simulink model "P2_0D_model_parametrized"  (R2023a)
settings: Solver=ode4  StartTime=0.0  StopTime=inf  FixedStep=Ts  RelTol=1e-3
model workspace (MAT data in the model file):
  Ts = Simulink.Parameter
  Ts.Value = 0.0005
  Ts.DataType = 'auto'
  Ts.Complexity = 'real'
  Ts.Dimensions = [1 1]
undefined symbols (not defined in the file or in its folder): data, HR, left_ventricle_R_wall, MLAP, MRAP, openloop
libraries: Vessel x42, simulink x2
(part 1 of 2)
settings Model: Creator=emanuele  LastModifiedBy=priya
settings DataIOCC: FinalStateName=final_simstate  InitialState=new_simstate  SaveFinalState=on  SaveOperatingPoint=on
settings OptimizationCC: ReuseModelBlockBuffer=off

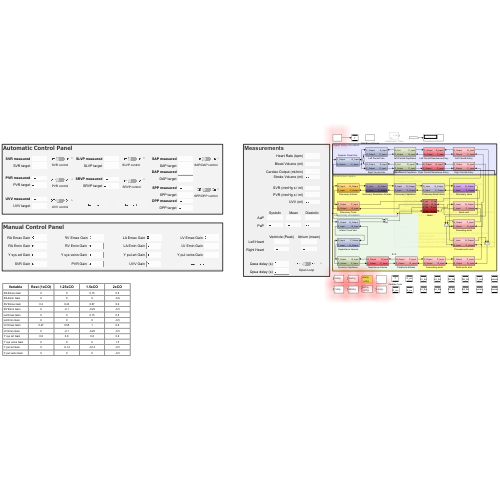
[thumbnail: Simulink's stored preview of the top-level diagram]
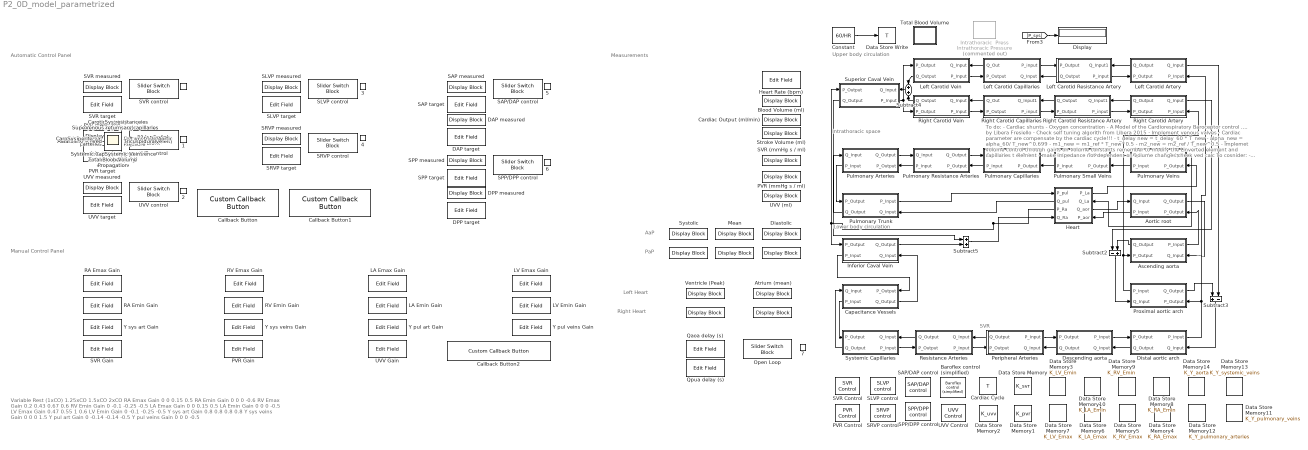
== system P2_0D_model_parametrized ==
  note: AaP
  note: Measurements
  note: Automatic Control Panel
  note: SVR
  note: To do:
      |
      | - Cardiac shunts
      | - Oxygen concentration
      | - A Model of the Cardiorespiratory  Baroceptor control .... by Libera Fresiello
      | - Check self tuning algorith from Libera 2015
      | - Implement venous valves
      | - Cardiac parameter are compensate by the cardiac cycle!!!
      |            - t_delay new = t_delay_60 * T_new
      |            - alpha_new = alpha_60/ T_new^0.699
      |            - m1_new = m1_ref * T_new^0.5
      |            - m2_new = m2_ref / T_new^0.5
      | - Implemet volume control through gains on volume constants
      | remember to modify the Linverted element and capillaries t element - make impedance
      | not dependent on volume changes
      |
      | check ved calc
      |
      | To cosnider:
      |
      | - Valves' Bernoulli resistance has to be divided by 100 or 1000. It strongly affects
      | the behaviour of the whole system
      | - The inductance and the resistances of the vessels do not change over time
      | - Reatime optimization  to patient ? like with smatwatch data (https://www.cardiacsense.com/wp-content/uploads/2019/10/2022_05_11_ENGLISH_WEBSITE.pdf).
      |
      | Ideas:
      |
      | - Patient specific optmisazion with smart watch, cloud server, etc foo prediction of???
      |   - High ematocrit level. Hypotension etc.
      | - Use locomotory data from patient during walking, incorporate it into the model,
      |   potentially demosntrate 1:1 coupling.
      | - maybe incorporate the metabolic consumpton too?
      | - Use MRI images of vasculature to derive geometrical parameters
      | - COmbine 0D model with 1 D model of specfic tract? check simvascular for ull ody model
      | - Black box for nils (protected model)
      |
      | Questions to Broomé:
      | - Do inductances and resistances change over time with vessel's radius?
      | - Having problem with allowing negative flow at the valves.
  note: Upper body circulation
  note: Intrathoracic space
  note: Lower body circulation
  note: Manual Control Panel
  note: PaP
  note: Left Heart
  note: Right Heart
  note: Variable
      | Rest (1xCO)
      | 1.25xCO
      | 1.5xCO
      | 2xCO
      |
      | RA Emax Gain
      | 0
      | 0
      | 0.15
      | 0.5
      |
      | RA Emin Gain
      | 0
      | 0
      | 0
      | -0.6
      |
      | RV Emax Gain
      | 0.2
      | 0.43
      | 0.67
      | 0.6
      |
      | RV Emin Gain
      | 0
      | -0.1
      | -0.25
      | -0.5
      |
      | LA Emax Gain
      | 0
      | 0
      | 0.15
      | 0.5
      |
      | LA Emin Gain
      | 0
      | 0
      | 0
      | -0.5
      |
      | LV Emax Gain
      | 0.47
      | 0.55
      | 1
      | 0.6
      |
      | LV Emin Gain
      | 0
      | -0.1
      | -0.25
      | -0.5
      |
      | Y sys art Gain
      | 0.8
      | 0.8
      | 0.8
      | 0.8
      |
      | Y sys veins Gain
      | 0
      | 0
      | 0
      | 1.5
      |
      | Y pul art Gain
      | 0
      | -0.14
      | -0.14
      | -0.5
      |
      | Y pul veins Gain
      | 0
      | 0
      | 0
      | -0.5
   {,3..7} (6 alike) : LampBlock  LabelPosition=Hide  Opacity=0.5
  "  " : DisplayBlock  LabelPosition=Hide  Format=Custom  Alignment=Left  Transparency=1  Layout=Fill available space  FormatString=%.2f
  "   " : DisplayBlock  LabelPosition=Hide  Format=Custom  Alignment=Left  Transparency=1  Layout=Fill available space  FormatString=%.2f
  "     " : DisplayBlock  LabelPosition=Hide  Format=Custom  Alignment=Left  Transparency=1  Layout=Fill available space  FormatString=%.2f
  "      " : DisplayBlock  LabelPosition=Hide  Format=Custom  Alignment=Left  Transparency=1  Layout=Fill available space  FormatString=%.2f
  "          " : DisplayBlock  LabelPosition=Hide  Format=Custom  Alignment=Left  Transparency=1  Layout=Fill available space  FormatString=%.2f
  " 1" : LampBlock  LabelPosition=Hide
  " 2" : LampBlock  LabelPosition=Hide
  Aortic root : Subsystem
      settings: PortSchema="{\"entries\":[{\"content\":{\"sides\":[{\"content\":{\"connectorIds\":[\"In1\",\"Out2\"]},\"type\":\"ConnectorPlacement.EquallySpacedRectSide\",\"uuid\":\"4620f5c1-12c0-4f29-952b-739216107ff5\"},{\"content\":{\"connectorIds\":[\"Out1\",\"In2\"],\"side\":\"RIGHT\"},\"type\":\"ConnectorPlacement.EquallySpacedRectSide\",\"uuid\":\"dda98628-74f0-4e08-ba9e-db399286a987\"},{\"content\":{\"connectorIds\":[],\"side\":\"TOP\"},\"type\":\"ConnectorPlacement.EquallySpacedRectSide\",\"uuid\":\"6ce998cb-1877-491b-b2c2-215d41cdcb23\"},{\"content\":{\"connectorIds\":[],\"side\":\"BOTTOM\"},\"type\":\"ConnectorPlacement.EquallySpacedRectSide\",\"uuid\":\"85207667-2600-4d53-af68-3471fed39a56\"}]},\"type\":\"ConnectorPlacement.EquallySpacedConnector\",\"uuid\":\"3b979ad0-f04d-4546-9a99-5921572b1183\"}],\"packageUris\":[\"http://schema.mathworks.com/mf0/Connector/R2020b\"],\"version\":\"1.0\"}"
  Ascending aorta : Subsystem  Description=asrwer
      settings: PortSchema="{\"entries\":[{\"content\":{\"sides\":[{\"content\":{\"connectorIds\":[\"Out2\",\"In1\"]},\"type\":\"ConnectorPlacement.EquallySpacedRectSide\",\"uuid\":\"4620f5c1-12c0-4f29-952b-739216107ff5\"},{\"content\":{\"connectorIds\":[\"Out1\",\"In2\"],\"side\":\"RIGHT\"},\"type\":\"ConnectorPlacement.EquallySpacedRectSide\",\"uuid\":\"dda98628-74f0-4e08-ba9e-db399286a987\"},{\"content\":{\"connectorIds\":[],\"side\":\"TOP\"},\"type\":\"ConnectorPlacement.EquallySpacedRectSide\",\"uuid\":\"6ce998cb-1877-491b-b2c2-215d41cdcb23\"},{\"content\":{\"connectorIds\":[],\"side\":\"BOTTOM\"},\"type\":\"ConnectorPlacement.EquallySpacedRectSide\",\"uuid\":\"dba296ee-e2cd-4942-9262-f71d521616c7\"}]},\"type\":\"ConnectorPlacement.EquallySpacedConnector\",\"uuid\":\"3b979ad0-f04d-4546-9a99-5921572b1183\"}],\"packageUris\":[\"http://schema.mathworks.com/mf0/Connector/R2020b\"],\"version\":\"1.0\"}"
  Atrium (mean) : DisplayBlock  LabelPosition=Hide  Format=Custom  Alignment=Left  Transparency=1  Layout=Fill available space  FormatString=%.2f
  Baroflex control (simplified) : Vessel/Baroflex control (simplified)  G_baro=0.04  P_target=92  T_target=60/72  onoff=off
      settings: SourceProductName=CVM
  Blood Volume (ml) : DisplayBlock  LabelPosition=Hide  Format=Custom  Alignment=Left  Transparency=1  Layout=Fill available space  FormatString=%.f
  Callback Button : CustomCallbackButton  Configuration="{\"components\":[{\"name\":\"BackgroundImageComponent\",\"settings\":{\"image\":{\"size\":[0,0],\"src\":\"default\",\"srcOrientation\":\"Right\"},\"position\":[0,0,1,1]}},{\"name\":\"ButtonStateComponent\",\"settings\":{\"buttonType\":\"momentary\",\"clickFcn\":\"coder.extrinsic('set_param')\\nset_param(['' bdroot '\\/SVR Control\\/Constant1'],'Value',sprintf('%d',0));\\nset_param(['' bdroot '\\/PVR Control\\/Constant1'],'Value',sprintf('%d',0));\\n\\nset_param(['' bdroot '\\/SLVP control\\/Constant1'],'Value',sprintf('%d',0));\\nset_param(['' bdroot '\\/SRVP control\\/Constant1'],'Value',sprintf('%d',0));\\n\\nset_param(['' bdroot '\\/SAP\\/\\/DAP control\\/Constant1'],'Value',sprintf('%d',0));\\nset_param(['' bdroot '\\/SPP\\/\\/DPP control\\/Constant1'],'Value',sprintf('%d',0));\\n\",\"onValue\":1,\"position\":[0,0,1,1],\"pressDelay\":\"500\",\"pressFcn\":\"\",\"repeatInterval\":\"0\",\"states\":[{\"horizontalAlignment\":\"center\",\"image\":{\"position\":[0,0,1,1],\"src\":\"default\",\"srcOrientation\":\"Right\"},\"label\":{\"color\":[0.01176470588,0.01176470588,0.01176470588,1],\"icon\":{\"size\":[0,0],\"src\":\"default\",\"srcOrientation\":\"Right\"},\"iconPlacement\":\"left\",\"text\":{\"content\":\"Turn off all\"}},\"labelOffset\":[0,0],\"verticalAlignment\":\"middle\"},{\"horizontalAlignment\":\"center\",\"image\":{\"position\":[0,0,1,1],\"src\":\"default\",\"srcOrientation\":\"Right\"},\"label\":{\"color\":[0.01176470588,0.01176470588,0.01176470588,1],\"icon\":{\"size\":[0,0],\"src\":\"default\",\"srcOrientation\":\"Right\"},\"iconPlacement\":\"left\",\"text\":{\"content\":\"Turn off all\"}},\"labelOffset\":[0,0],\"verticalAlignment\":\"middle\"},{\"horizontalAlignment\":\"center\",\"image\":{\"position\":[0,0,1,1],\"src\":\"default\",\"srcOrientation\":\"Right\"},\"label\":{\"color\":[0.01176470588,0.01176470588,0.01176470588,1],\"icon\":{\"size\":[0,0],\"src\":\"default\",\"srcOrientation\":\"Right\"},\"iconPlacement\":\"left\",\"text\":{\"content\":\"Turn off all\"}},\"labelOffset\":[0,0],\"verticalAlignment\":\"middle\"},{\"horizontalAlignment\":\"center\",\"image\":{\"position\":[0,0,1,1],\"src\":\"default\",\"srcOrientation\":\"Right\"},\"label\":{\"color\":[0.01176470588,0.01176470588,0.01176470588,1],\"icon\":{\"size\":[0,0],\"src\":\"default\",\"srcOrientation\":\"Right\"},\"iconPlacement\":\"left\",\"text\":{\"content\":\"Turn off all\"}},\"labelOffset\":[0,0],\"verticalAlignment\":\"middle\"}]}},{\"name\":\"ForegroundImageComponent\",\"settings\":{\"image\":{\"size\":[0,0],\"src\":\"default\",\"srcOrientation\":\"Right\"},\"isForeground\":1,\"position\":[0,0,1,1]}}],\"settings\":{\"BindingType\":\"standalone\",\"backgroundColor\":[244,244,244,1],\"backgroundOffset\":0.2,\"backgroundOpacity\":1,\"fixedAspectRatio\":\"off\",\"foregroundColor\":[0.01176470588,0.01176470588,0.01176470588,1],\"migratedFromLegacy\":true,\"useBackgroundColor\":true,\"variant\":\"callback\",\"version\":\"R2023a\"},\"type\":\"Button\"}"  CustomBackgroundColor="{\"color\":[0.9568627451,0.9568627451,0.9568627451],\"show\":true}"
  Callback Button1 : CustomCallbackButton  Configuration="{\"components\":[{\"name\":\"BackgroundImageComponent\",\"settings\":{\"image\":{\"size\":[0,0],\"src\":\"default\",\"srcOrientation\":\"Right\"},\"position\":[0,0,1,1]}},{\"name\":\"ButtonStateComponent\",\"settings\":{\"buttonType\":\"momentary\",\"clickFcn\":\"coder.extrinsic('set_param')\\nset_param(['' bdroot '\\/SVR Control\\/Constant1'],'Value',sprintf('%d',1));\\nset_param(['' bdroot '\\/PVR Control\\/Constant1'],'Value',sprintf('%d',1));\\n\\nset_param(['' bdroot '\\/SLVP control\\/Constant1'],'Value',sprintf('%d',1));\\nset_param(['' bdroot '\\/SRVP control\\/Constant1'],'Value',sprintf('%d',1));\\n\\nset_param(['' bdroot '\\/SAP\\/\\/DAP control\\/Constant1'],'Value',sprintf('%d',1));\\nset_param(['' bdroot '\\/SPP\\/\\/DPP control\\/Constant1'],'Value',sprintf('%d',1));\\n\",\"onValue\":1,\"position\":[0,0,1,1],\"pressDelay\":\"500\",\"pressFcn\":\"\",\"repeatInterval\":\"0\",\"states\":[{\"horizontalAlignment\":\"center\",\"image\":{\"position\":[0,0,1,1],\"src\":\"default\",\"srcOrientation\":\"Right\"},\"label\":{\"color\":[0.01176470588,0.01176470588,0.01176470588,1],\"icon\":{\"size\":[0,0],\"src\":\"default\",\"srcOrientation\":\"Right\"},\"iconPlacement\":\"left\",\"text\":{\"content\":\"Turn on all\"}},\"labelOffset\":[0,0],\"verticalAlignment\":\"middle\"},{\"horizontalAlignment\":\"center\",\"image\":{\"position\":[0,0,1,1],\"src\":\"default\",\"srcOrientation\":\"Right\"},\"label\":{\"color\":[0.01176470588,0.01176470588,0.01176470588,1],\"icon\":{\"size\":[0,0],\"src\":\"default\",\"srcOrientation\":\"Right\"},\"iconPlacement\":\"left\",\"text\":{\"content\":\"Turn on all\"}},\"labelOffset\":[0,0],\"verticalAlignment\":\"middle\"},{\"horizontalAlignment\":\"center\",\"image\":{\"position\":[0,0,1,1],\"src\":\"default\",\"srcOrientation\":\"Right\"},\"label\":{\"color\":[0.01176470588,0.01176470588,0.01176470588,1],\"icon\":{\"size\":[0,0],\"src\":\"default\",\"srcOrientation\":\"Right\"},\"iconPlacement\":\"left\",\"text\":{\"content\":\"Turn on all\"}},\"labelOffset\":[0,0],\"verticalAlignment\":\"middle\"},{\"horizontalAlignment\":\"center\",\"image\":{\"position\":[0,0,1,1],\"src\":\"default\",\"srcOrientation\":\"Right\"},\"label\":{\"color\":[0.01176470588,0.01176470588,0.01176470588,1],\"icon\":{\"size\":[0,0],\"src\":\"default\",\"srcOrientation\":\"Right\"},\"iconPlacement\":\"left\",\"text\":{\"content\":\"Turn on all\"}},\"labelOffset\":[0,0],\"verticalAlignment\":\"middle\"}]}},{\"name\":\"ForegroundImageComponent\",\"settings\":{\"image\":{\"size\":[0,0],\"src\":\"default\",\"srcOrientation\":\"Right\"},\"isForeground\":1,\"position\":[0,0,1,1]}}],\"settings\":{\"BindingType\":\"standalone\",\"backgroundColor\":[244,244,244,1],\"backgroundOffset\":0.2,\"backgroundOpacity\":1,\"fixedAspectRatio\":\"off\",\"foregroundColor\":[0.01176470588,0.01176470588,0.01176470588,1],\"migratedFromLegacy\":true,\"useBackgroundColor\":true,\"variant\":\"callback\",\"version\":\"R2023a\"},\"type\":\"Button\"}"  CustomBackgroundColor="{\"color\":[0.9568627451,0.9568627451,0.9568627451],\"show\":true}"
  Callback Button2 : CustomCallbackButton  Configuration="{\"components\":[{\"name\":\"BackgroundImageComponent\",\"settings\":{\"image\":{\"size\":[0,0],\"src\":\"default\",\"srcOrientation\":\"Right\"},\"position\":[0,0,1,1]}},{\"name\":\"ButtonStateComponent\",\"settings\":{\"buttonType\":\"momentary\",\"clickFcn\":\"coder.extrinsic('set_param')\\nset_param(['' bdroot '\\/SVR Control\\/K_svr'],'Value',sprintf('%d',0));\\nset_param(['' bdroot '\\/PVR Control\\/K_pvr'],'Value',sprintf('%d',0));\\n\\nset_param(['' bdroot '\\/SLVP control\\/K_LV_Emax'],'Value',sprintf('%d',0));\\nset_param(['' bdroot '\\/SLVP control\\/K_LV_Emin'],'Value',sprintf('%d',0));\\nset_param(['' bdroot '\\/SLVP control\\/K_LA_Emax'],'Value',sprintf('%d',0));\\nset_param(['' bdroot '\\/SLVP control\\/K_LA_Emin'],'Value',sprintf('%d',0));\\n\\nset_param(['' bdroot '\\/SRVP control\\/K_RV_Emax'],'Value',sprintf('%d',0));\\nset_param(['' bdroot '\\/SRVP control\\/K_RV_Emin'],'Value',sprintf('%d',0));\\nset_param(['' bdroot '\\/SRVP control\\/K_RA_Emax'],'Value',sprintf('%d',0));\\nset_param(['' bdroot '\\/SRVP control\\/K_RA_Emin'],'Value',sprintf('%d',0));\\n\\nset_param(['' bdroot '\\/SAP\\/\\/DAP control\\/K_Y_aorta'],'Value',sprintf('%d',0));\\nset_param(['' bdroot '\\/SAP\\/\\/DAP control\\/K_Y_systemic_veins'],'Value',sprintf('%d',0));\\n\\nset_param(['' bdroot '\\/SPP\\/\\/DPP control\\/K_Y_pulmonary_arteries'],'Value',sprintf('%d',0));\\nset_param(['' bdroot '\\/SPP\\/\\/DPP control\\/K_Y_pulmonary_veins'],'Value',sprintf('%d',0));\\n\\n\",\"onValue\":1,\"position\":[0,0,1,1],\"pressDelay\":\"500\",\"pressFcn\":\"\",\"repeatInterval\":\"0\",\"states\":[{\"horizontalAlignment\":\"center\",\"image\":{\"position\":[0,0,1,1],\"src\":\"default\",\"srcOrientation\":\"Right\"},\"label\":{\"color\":[0.01176470588,0.01176470588,0.01176470588,1],\"icon\":{\"size\":[0,0],\"src\":\"default\",\"srcOrientation\":\"Right\"},\"iconPlacement\":\"left\",\"text\":{\"content\":\"Reset Gains\"}},\"labelOffset\":[0,0],\"verticalAlignment\":\"middle\"},{\"horizontalAlignment\":\"center\",\"image\":{\"position\":[0,0,1,1],\"src\":\"default\",\"srcOrientation\":\"Right\"},\"label\":{\"color\":[0.01176470588,0.01176470588,0.01176470588,1],\"icon\":{\"size\":[0,0],\"src\":\"default\",\"srcOrientation\":\"Right\"},\"iconPlacement\":\"left\",\"text\":{\"content\":\"Reset Gains\"}},\"labelOffset\":[0,0],\"verticalAlignment\":\"middle\"},{\"horizontalAlignment\":\"center\",\"image\":{\"position\":[0,0,1,1],\"src\":\"default\",\"srcOrientation\":\"Right\"},\"label\":{\"color\":[0.01176470588,0.01176470588,0.01176470588,1],\"icon\":{\"size\":[0,0],\"src\":\"default\",\"srcOrientation\":\"Right\"},\"iconPlacement\":\"left\",\"text\":{\"content\":\"Reset Gains\"}},\"labelOffset\":[0,0],\"verticalAlignment\":\"middle\"},{\"horizontalAlignment\":\"center\",\"image\":{\"position\":[0,0,1,1],\"src\":\"default\",\"srcOrientation\":\"Right\"},\"label\":{\"color\":[0.01176470588,0.01176470588,0.01176470588,1],\"icon\":{\"size\":[0,0],\"src\":\"default\",\"srcOrientation\":\"Right\"},\"iconPlacement\":\"left\",\"text\":{\"content\":\"Reset Gains\"}},\"labelOffset\":[0,0],\"verticalAlignment\":\"middle\"}]}},{\"name\":\"ForegroundImageComponent\",\"settings\":{\"image\":{\"size\":[0,0],\"src\":\"default\",\"srcOrientation\":\"Right\"},\"isForeground\":1,\"position\":[0,0,1,1]}}],\"settings\":{\"BindingType\":\"standalone\",\"backgroundColor\":[244,244,244,1],\"backgroundOffset\":0.2,\"backgroundOpacity\":1,\"fixedAspectRatio\":\"off\",\"foregroundColor\":[0.01176470588,0.01176470588,0.01176470588,1],\"migratedFromLegacy\":true,\"useBackgroundColor\":true,\"variant\":\"callback\",\"version\":\"R2023a\"},\"type\":\"Button\"}"  CustomBackgroundColor="{\"color\":[0.9568627451,0.9568627451,0.9568627451],\"show\":true}"
  Capacitance Vessels : Subsystem  Description=asrwer
      settings: PortSchema="{\"entries\":[{\"content\":{\"sides\":[{\"content\":{\"connectorIds\":[\"In1\",\"Out2\"]},\"type\":\"ConnectorPlacement.EquallySpacedRectSide\",\"uuid\":\"4620f5c1-12c0-4f29-952b-739216107ff5\"},{\"content\":{\"connectorIds\":[\"In2\",\"Out1\"],\"side\":\"RIGHT\"},\"type\":\"ConnectorPlacement.EquallySpacedRectSide\",\"uuid\":\"dda98628-74f0-4e08-ba9e-db399286a987\"},{\"content\":{\"connectorIds\":[],\"side\":\"TOP\"},\"type\":\"ConnectorPlacement.EquallySpacedRectSide\",\"uuid\":\"6ce998cb-1877-491b-b2c2-215d41cdcb23\"},{\"content\":{\"connectorIds\":[],\"side\":\"BOTTOM\"},\"type\":\"ConnectorPlacement.EquallySpacedRectSide\",\"uuid\":\"722bc419-c275-4c63-b409-b29152115373\"}]},\"type\":\"ConnectorPlacement.EquallySpacedConnector\",\"uuid\":\"3b979ad0-f04d-4546-9a99-5921572b1183\"}],\"packageUris\":[\"http://schema.mathworks.com/mf0/Connector/R2020b\"],\"version\":\"1.0\"}"
  Cardiac Cycle : DataStoreMemory  DataStoreName=T  WriteAfterWriteMsg=warning  InitialValue=1  ShowAdditionalParam=off  OutMin=0  OutMax=1000
  Cardiac Output (ml/min) : DisplayBlock  LabelPosition=Hide  Format=Custom  Alignment=Left  Transparency=1  Layout=Fill available space  FormatString=%.f
  Constant : Constant  Value=60/HR
  DAP measured : DisplayBlock  LabelPosition=Hide  Format=Custom  Alignment=Left  Transparency=1  Layout=Fill available space  FormatString=%.2f
  DAP target : EditField  LabelPosition=Hide  ShowInitialText=on  Alignment=Left
  DPP measured : DisplayBlock  LabelPosition=Hide  Format=Custom  Alignment=Left  Transparency=1  Layout=Fill available space  FormatString=%.2f
  DPP target : EditField  LabelPosition=Hide  ShowInitialText=on  Alignment=Left
  Data Store Memory : DataStoreMemory  DataStoreName=K_svr  WriteAfterWriteMsg=warning  ShowAdditionalParam=off
  Data Store Memory1 : DataStoreMemory  DataStoreName=K_pvr  WriteAfterWriteMsg=warning  ShowAdditionalParam=off
  Data Store Memory10 : DataStoreMemory  DataStoreName=K_LA_Emin  WriteAfterWriteMsg=warning  ShowAdditionalParam=off
  Data Store Memory11 : DataStoreMemory  DataStoreName=K_Y_pulmonary_veins  WriteAfterWriteMsg=warning  ShowAdditionalParam=off
  Data Store Memory12 : DataStoreMemory  DataStoreName=K_Y_pulmonary_arteries  WriteAfterWriteMsg=warning  ShowAdditionalParam=off
  Data Store Memory13 : DataStoreMemory  DataStoreName=K_Y_systemic_veins  WriteAfterWriteMsg=warning  ShowAdditionalParam=off
  Data Store Memory14 : DataStoreMemory  DataStoreName=K_Y_aorta  WriteAfterWriteMsg=warning  ShowAdditionalParam=off
  Data Store Memory2 : DataStoreMemory  DataStoreName=K_uvv  WriteAfterWriteMsg=warning  ShowAdditionalParam=off
  Data Store Memory3 : DataStoreMemory  DataStoreName=K_LV_Emin  WriteAfterWriteMsg=warning  ShowAdditionalParam=off
  Data Store Memory4 : DataStoreMemory  DataStoreName=K_RA_Emax  WriteAfterWriteMsg=warning  ShowAdditionalParam=off
  Data Store Memory5 : DataStoreMemory  DataStoreName=K_RV_Emax  WriteAfterWriteMsg=warning  ShowAdditionalParam=off
  Data Store Memory6 : DataStoreMemory  DataStoreName=K_LA_Emax  WriteAfterWriteMsg=warning  ShowAdditionalParam=off
  Data Store Memory7 : DataStoreMemory  DataStoreName=K_LV_Emax  WriteAfterWriteMsg=warning  ShowAdditionalParam=off
  Data Store Memory8 : DataStoreMemory  DataStoreName=K_RA_Emin  WriteAfterWriteMsg=warning  ShowAdditionalParam=off
  Data Store Memory9 : DataStoreMemory  DataStoreName=K_RV_Emin  WriteAfterWriteMsg=warning  ShowAdditionalParam=off
  Data Store Write : DataStoreWrite  DataStoreName=T  IndexOptions=Index vector (dialog)  Indices=1  OutputSizes=1
  Descending aorta : Subsystem  Description=asrwer
      settings: PortSchema="{\"entries\":[{\"content\":{\"sides\":[{\"content\":{\"connectorIds\":[\"In1\",\"Out2\"]},\"type\":\"ConnectorPlacement.EquallySpacedRectSide\",\"uuid\":\"4620f5c1-12c0-4f29-952b-739216107ff5\"},{\"content\":{\"connectorIds\":[\"Out1\",\"In2\"],\"side\":\"RIGHT\"},\"type\":\"ConnectorPlacement.EquallySpacedRectSide\",\"uuid\":\"dda98628-74f0-4e08-ba9e-db399286a987\"},{\"content\":{\"connectorIds\":[],\"side\":\"TOP\"},\"type\":\"ConnectorPlacement.EquallySpacedRectSide\",\"uuid\":\"6ce998cb-1877-491b-b2c2-215d41cdcb23\"},{\"content\":{\"connectorIds\":[],\"side\":\"BOTTOM\"},\"type\":\"ConnectorPlacement.EquallySpacedRectSide\",\"uuid\":\"98e366c2-00e2-468b-b3a5-0ce1b16c883f\"}]},\"type\":\"ConnectorPlacement.EquallySpacedConnector\",\"uuid\":\"3b979ad0-f04d-4546-9a99-5921572b1183\"}],\"packageUris\":[\"http://schema.mathworks.com/mf0/Connector/R2020b\"],\"version\":\"1.0\"}"
  Diastolic : DisplayBlock  LabelPosition=Hide  Format=Custom  Alignment=Left  Transparency=1  Layout=Fill available space  FormatString=%.2f
  Display : Display
  Distal aortic arch : Subsystem  Description=asrwer
      settings: PortSchema="{\"entries\":[{\"content\":{\"sides\":[{\"content\":{\"connectorIds\":[\"In1\",\"Out2\"]},\"type\":\"ConnectorPlacement.EquallySpacedRectSide\",\"uuid\":\"4620f5c1-12c0-4f29-952b-739216107ff5\"},{\"content\":{\"connectorIds\":[\"Out1\",\"In2\"],\"side\":\"RIGHT\"},\"type\":\"ConnectorPlacement.EquallySpacedRectSide\",\"uuid\":\"dda98628-74f0-4e08-ba9e-db399286a987\"},{\"content\":{\"connectorIds\":[],\"side\":\"TOP\"},\"type\":\"ConnectorPlacement.EquallySpacedRectSide\",\"uuid\":\"6ce998cb-1877-491b-b2c2-215d41cdcb23\"},{\"content\":{\"connectorIds\":[],\"side\":\"BOTTOM\"},\"type\":\"ConnectorPlacement.EquallySpacedRectSide\",\"uuid\":\"1f1286b1-33d8-470d-99d1-3841bccf9133\"}]},\"type\":\"ConnectorPlacement.EquallySpacedConnector\",\"uuid\":\"3b979ad0-f04d-4546-9a99-5921572b1183\"}],\"packageUris\":[\"http://schema.mathworks.com/mf0/Connector/R2020b\"],\"version\":\"1.0\"}"
  Heart : Subsystem  Description=asrwer
      settings: PortSchema="{\"entries\":[{\"content\":{\"sides\":[{\"content\":{\"connectorIds\":[\"In1\",\"Out3\",\"Out4\",\"In2\"]},\"type\":\"ConnectorPlacement.EquallySpacedRectSide\",\"uuid\":\"95824f71-698a-4f4d-a993-6df26fe534d7\"},{\"content\":{\"connectorIds\":[\"Out1\",\"In3\",\"Out2\",\"In4\"],\"side\":\"RIGHT\"},\"type\":\"ConnectorPlacement.EquallySpacedRectSide\",\"uuid\":\"a8959a41-c68c-4f70-a35f-cb85dc600e61\"},{\"content\":{\"connectorIds\":[],\"side\":\"TOP\"},\"type\":\"ConnectorPlacement.EquallySpacedRectSide\",\"uuid\":\"0158d717-51c0-4653-88b6-d7632d8acf9b\"},{\"content\":{\"connectorIds\":[],\"side\":\"BOTTOM\"},\"type\":\"ConnectorPlacement.EquallySpacedRectSide\",\"uuid\":\"36b7b652-46be-43bf-a0da-22ec9d4b557c\"}]},\"type\":\"ConnectorPlacement.EquallySpacedConnector\",\"uuid\":\"7f917747-c70e-4597-9ded-e790c0b0e5f8\"}],\"packageUris\":[\"http://schema.mathworks.com/mf0/Connector/R2020b\"],\"version\":\"1.0\"}"
  Heart Rate (bpm) : EditField  LabelPosition=Hide  ShowInitialText=on  Alignment=Left
  Inferior Caval Vein : Subsystem  Description=asrwer
      settings: PortSchema="{\"entries\":[{\"content\":{\"sides\":[{\"content\":{\"connectorIds\":[\"In1\",\"Out2\"]},\"type\":\"ConnectorPlacement.EquallySpacedRectSide\",\"uuid\":\"4620f5c1-12c0-4f29-952b-739216107ff5\"},{\"content\":{\"connectorIds\":[\"Out1\",\"In2\"],\"side\":\"RIGHT\"},\"type\":\"ConnectorPlacement.EquallySpacedRectSide\",\"uuid\":\"dda98628-74f0-4e08-ba9e-db399286a987\"},{\"content\":{\"connectorIds\":[],\"side\":\"TOP\"},\"type\":\"ConnectorPlacement.EquallySpacedRectSide\",\"uuid\":\"6ce998cb-1877-491b-b2c2-215d41cdcb23\"},{\"content\":{\"connectorIds\":[],\"side\":\"BOTTOM\"},\"type\":\"ConnectorPlacement.EquallySpacedRectSide\",\"uuid\":\"6fb320e2-add0-4ab2-8fb4-43aaa029b4e4\"}]},\"type\":\"ConnectorPlacement.EquallySpacedConnector\",\"uuid\":\"3b979ad0-f04d-4546-9a99-5921572b1183\"}],\"packageUris\":[\"http://schema.mathworks.com/mf0/Connector/R2020b\"],\"version\":\"1.0\"}"
  Intrathoracic  Press : Vessel/Intrathoracic Pressure  Commented=on  t_ins=2  t_exp=3  p_ita=1.8  p_itb=-5.5
      settings: SourceProductName=CVM
  LA Emax Gain : EditField  LabelPosition=Hide  ShowInitialText=on  Alignment=Left
  LA Emin Gain : EditField  LabelPosition=Hide  ShowInitialText=on  Alignment=Left
  LV Emax Gain : EditField  LabelPosition=Hide  ShowInitialText=on  Alignment=Left
  LV Emin Gain : EditField  LabelPosition=Hide  ShowInitialText=on  Alignment=Left
  Left Carotid Artery : Subsystem  Description=asrwer
      settings: PortSchema="{\"entries\":[{\"content\":{\"sides\":[{\"content\":{\"connectorIds\":[\"Out2\",\"In1\"]},\"type\":\"ConnectorPlacement.EquallySpacedRectSide\",\"uuid\":\"4620f5c1-12c0-4f29-952b-739216107ff5\"},{\"content\":{\"connectorIds\":[\"Out1\",\"In2\"],\"side\":\"RIGHT\"},\"type\":\"ConnectorPlacement.EquallySpacedRectSide\",\"uuid\":\"dda98628-74f0-4e08-ba9e-db399286a987\"},{\"content\":{\"connectorIds\":[],\"side\":\"TOP\"},\"type\":\"ConnectorPlacement.EquallySpacedRectSide\",\"uuid\":\"6ce998cb-1877-491b-b2c2-215d41cdcb23\"},{\"content\":{\"connectorIds\":[],\"side\":\"BOTTOM\"},\"type\":\"ConnectorPlacement.EquallySpacedRectSide\",\"uuid\":\"47027a70-0169-4a10-9704-3eebb5be1f94\"}]},\"type\":\"ConnectorPlacement.EquallySpacedConnector\",\"uuid\":\"3b979ad0-f04d-4546-9a99-5921572b1183\"}],\"packageUris\":[\"http://schema.mathworks.com/mf0/Connector/R2020b\"],\"version\":\"1.0\"}"
  Left Carotid Capillaries : Subsystem  Description=asrwer
      settings: PortSchema="{\"entries\":[{\"content\":{\"sides\":[{\"content\":{\"connectorIds\":[\"Out2\",\"In1\"]},\"type\":\"ConnectorPlacement.EquallySpacedRectSide\",\"uuid\":\"4620f5c1-12c0-4f29-952b-739216107ff5\"},{\"content\":{\"connectorIds\":[\"Out1\",\"In2\"],\"side\":\"RIGHT\"},\"type\":\"ConnectorPlacement.EquallySpacedRectSide\",\"uuid\":\"dda98628-74f0-4e08-ba9e-db399286a987\"},{\"content\":{\"connectorIds\":[],\"side\":\"TOP\"},\"type\":\"ConnectorPlacement.EquallySpacedRectSide\",\"uuid\":\"6ce998cb-1877-491b-b2c2-215d41cdcb23\"},{\"content\":{\"connectorIds\":[],\"side\":\"BOTTOM\"},\"type\":\"ConnectorPlacement.EquallySpacedRectSide\",\"uuid\":\"55c6bb06-9ed0-4db0-b546-e99e0ef08408\"}]},\"type\":\"ConnectorPlacement.EquallySpacedConnector\",\"uuid\":\"3b979ad0-f04d-4546-9a99-5921572b1183\"}],\"packageUris\":[\"http://schema.mathworks.com/mf0/Connector/R2020b\"],\"version\":\"1.0\"}"
  Left Carotid Resistance Artery : Subsystem  Description=asrwer
      settings: PortSchema="{\"entries\":[{\"content\":{\"sides\":[{\"content\":{\"connectorIds\":[\"In1\",\"Out2\"]},\"type\":\"ConnectorPlacement.EquallySpacedRectSide\",\"uuid\":\"d2373093-dd34-4525-a7d5-a44f41a4186f\"},{\"content\":{\"connectorIds\":[\"In2\",\"Out1\"],\"side\":\"RIGHT\"},\"type\":\"ConnectorPlacement.EquallySpacedRectSide\",\"uuid\":\"d0ccba4c-fde8-4729-94ab-e77f6e90fb41\"},{\"content\":{\"connectorIds\":[],\"side\":\"TOP\"},\"type\":\"ConnectorPlacement.EquallySpacedRectSide\",\"uuid\":\"7f992dfa-60d0-4d20-a39d-6e17177f43eb\"},{\"content\":{\"connectorIds\":[],\"side\":\"BOTTOM\"},\"type\":\"ConnectorPlacement.EquallySpacedRectSide\",\"uuid\":\"2327e57f-2f10-4013-b93e-75b24ceebb4e\"}]},\"type\":\"ConnectorPlacement.EquallySpacedConnector\",\"uuid\":\"d7eff068-f330-41b8-9147-abcbffe8f160\"}],\"packageUris\":[\"http://schema.mathworks.com/mf0/Connector/R2020b\"],\"version\":\"1.0\"}"
  Left Carotid Vein : Subsystem  Description=asrwer
      settings: PortSchema="{\"entries\":[{\"content\":{\"sides\":[{\"content\":{\"connectorIds\":[\"In1\",\"Out2\"]},\"type\":\"ConnectorPlacement.EquallySpacedRectSide\",\"uuid\":\"4620f5c1-12c0-4f29-952b-739216107ff5\"},{\"content\":{\"connectorIds\":[\"In2\",\"Out1\"],\"side\":\"RIGHT\"},\"type\":\"ConnectorPlacement.EquallySpacedRectSide\",\"uuid\":\"dda98628-74f0-4e08-ba9e-db399286a987\"},{\"content\":{\"connectorIds\":[],\"side\":\"TOP\"},\"type\":\"ConnectorPlacement.EquallySpacedRectSide\",\"uuid\":\"6ce998cb-1877-491b-b2c2-215d41cdcb23\"}]},\"type\":\"ConnectorPlacement.EquallySpacedConnector\",\"uuid\":\"3b979ad0-f04d-4546-9a99-5921572b1183\"}],\"packageUris\":[\"http://schema.mathworks.com/mf0/Connector/R2020b\"],\"version\":\"1.0\"}"
  Mean : DisplayBlock  LabelPosition=Hide  Format=Custom  Alignment=Left  Transparency=1  Layout=Fill available space  FormatString=%.2f
  Open Loop : SliderSwitchBlock  LabelPosition=Hide
      settings: Values={{'Off', 'On'}, [0 1]}
  PVR (mmHg s / ml) : DisplayBlock  LabelPosition=Hide  Format=Custom  Alignment=Left  Transparency=1  Layout=Fill available space  FormatString=%.2f
  PVR Control : Vessel/PVR Control  PVR_0=PVR  onoff=off
      link override Constant1: Value=0
      link override K_pvr: Value=0
      link override PID Controller: P=0.2  I=0.2
      settings: SourceProductName=CVM
  PVR Gain : EditField  LabelPosition=Hide  ShowInitialText=on  Alignment=Left
  PVR control : SliderSwitchBlock  LabelPosition=Hide
      settings: Values={{'Off', 'On'}, [0 1]}
  PVR measured : DisplayBlock  LabelPosition=Hide  Format=Custom  Alignment=Left  Transparency=1  Layout=Fill available space  FormatString=%.2f
  PVR target : EditField  LabelPosition=Hide  ShowInitialText=on  Alignment=Left
  Peripheral Arteries : Subsystem  Description=asrwer
      settings: PortSchema="{\"entries\":[{\"content\":{\"sides\":[{\"content\":{\"connectorIds\":[\"Out2\",\"In1\"]},\"type\":\"ConnectorPlacement.EquallySpacedRectSide\",\"uuid\":\"4620f5c1-12c0-4f29-952b-739216107ff5\"},{\"content\":{\"connectorIds\":[\"Out1\",\"In2\"],\"side\":\"RIGHT\"},\"type\":\"ConnectorPlacement.EquallySpacedRectSide\",\"uuid\":\"dda98628-74f0-4e08-ba9e-db399286a987\"},{\"content\":{\"connectorIds\":[],\"side\":\"TOP\"},\"type\":\"ConnectorPlacement.EquallySpacedRectSide\",\"uuid\":\"6ce998cb-1877-491b-b2c2-215d41cdcb23\"}]},\"type\":\"ConnectorPlacement.EquallySpacedConnector\",\"uuid\":\"3b979ad0-f04d-4546-9a99-5921572b1183\"}],\"packageUris\":[\"http://schema.mathworks.com/mf0/Connector/R2020b\"],\"version\":\"1.0\"}"
  Proximal aortic arch : Subsystem  Description=asrwer
      settings: PortSchema="{\"entries\":[{\"content\":{\"sides\":[{\"content\":{\"connectorIds\":[\"Out2\",\"In1\"]},\"type\":\"ConnectorPlacement.EquallySpacedRectSide\",\"uuid\":\"4620f5c1-12c0-4f29-952b-739216107ff5\"},{\"content\":{\"connectorIds\":[\"Out1\",\"In2\"],\"side\":\"RIGHT\"},\"type\":\"ConnectorPlacement.EquallySpacedRectSide\",\"uuid\":\"dda98628-74f0-4e08-ba9e-db399286a987\"},{\"content\":{\"connectorIds\":[],\"side\":\"TOP\"},\"type\":\"ConnectorPlacement.EquallySpacedRectSide\",\"uuid\":\"6ce998cb-1877-491b-b2c2-215d41cdcb23\"},{\"content\":{\"connectorIds\":[],\"side\":\"BOTTOM\"},\"type\":\"ConnectorPlacement.EquallySpacedRectSide\",\"uuid\":\"6fdba645-d59c-41ca-a267-e7525d3dc150\"}]},\"type\":\"ConnectorPlacement.EquallySpacedConnector\",\"uuid\":\"3b979ad0-f04d-4546-9a99-5921572b1183\"}],\"packageUris\":[\"http://schema.mathworks.com/mf0/Connector/R2020b\"],\"version\":\"1.0\"}"
  Pulmonary Arteries : Subsystem  Description=asrwer
      settings: PortSchema="{\"entries\":[{\"content\":{\"sides\":[{\"content\":{\"connectorIds\":[\"In1\",\"Out2\"]},\"type\":\"ConnectorPlacement.EquallySpacedRectSide\",\"uuid\":\"4620f5c1-12c0-4f29-952b-739216107ff5\"},{\"content\":{\"connectorIds\":[\"Out1\",\"In2\"],\"side\":\"RIGHT\"},\"type\":\"ConnectorPlacement.EquallySpacedRectSide\",\"uuid\":\"dda98628-74f0-4e08-ba9e-db399286a987\"},{\"content\":{\"connectorIds\":[],\"side\":\"TOP\"},\"type\":\"ConnectorPlacement.EquallySpacedRectSide\",\"uuid\":\"6ce998cb-1877-491b-b2c2-215d41cdcb23\"},{\"content\":{\"connectorIds\":[],\"side\":\"BOTTOM\"},\"type\":\"ConnectorPlacement.EquallySpacedRectSide\",\"uuid\":\"b2958bd4-f048-459f-a2a1-00e3322b7fc4\"}]},\"type\":\"ConnectorPlacement.EquallySpacedConnector\",\"uuid\":\"3b979ad0-f04d-4546-9a99-5921572b1183\"}],\"packageUris\":[\"http://schema.mathworks.com/mf0/Connector/R2020b\"],\"version\":\"1.0\"}"
  Pulmonary Capillaries : Subsystem  Description=asrwer
      settings: PortSchema="{\"entries\":[{\"content\":{\"sides\":[{\"content\":{\"connectorIds\":[\"In1\",\"Out2\"]},\"type\":\"ConnectorPlacement.EquallySpacedRectSide\",\"uuid\":\"4620f5c1-12c0-4f29-952b-739216107ff5\"},{\"content\":{\"connectorIds\":[\"Out1\",\"In2\"],\"side\":\"RIGHT\"},\"type\":\"ConnectorPlacement.EquallySpacedRectSide\",\"uuid\":\"dda98628-74f0-4e08-ba9e-db399286a987\"},{\"content\":{\"connectorIds\":[],\"side\":\"TOP\"},\"type\":\"ConnectorPlacement.EquallySpacedRectSide\",\"uuid\":\"6ce998cb-1877-491b-b2c2-215d41cdcb23\"},{\"content\":{\"connectorIds\":[],\"side\":\"BOTTOM\"},\"type\":\"ConnectorPlacement.EquallySpacedRectSide\",\"uuid\":\"a5d17b15-fcf6-4394-a6ba-03d04e8a34a2\"}]},\"type\":\"ConnectorPlacement.EquallySpacedConnector\",\"uuid\":\"3b979ad0-f04d-4546-9a99-5921572b1183\"}],\"packageUris\":[\"http://schema.mathworks.com/mf0/Connector/R2020b\"],\"version\":\"1.0\"}"
  Pulmonary Resistance Arteries : Subsystem  Description=asrwer
      settings: PortSchema="{\"entries\":[{\"content\":{\"sides\":[{\"content\":{\"connectorIds\":[\"In1\",\"Out2\"]},\"type\":\"ConnectorPlacement.EquallySpacedRectSide\",\"uuid\":\"4620f5c1-12c0-4f29-952b-739216107ff5\"},{\"content\":{\"connectorIds\":[\"Out1\",\"In2\"],\"side\":\"RIGHT\"},\"type\":\"ConnectorPlacement.EquallySpacedRectSide\",\"uuid\":\"dda98628-74f0-4e08-ba9e-db399286a987\"},{\"content\":{\"connectorIds\":[],\"side\":\"TOP\"},\"type\":\"ConnectorPlacement.EquallySpacedRectSide\",\"uuid\":\"6ce998cb-1877-491b-b2c2-215d41cdcb23\"},{\"content\":{\"connectorIds\":[],\"side\":\"BOTTOM\"},\"type\":\"ConnectorPlacement.EquallySpacedRectSide\",\"uuid\":\"a4fcb2d7-d0b3-4cd9-b62c-2f8a41b0f34e\"}]},\"type\":\"ConnectorPlacement.EquallySpacedConnector\",\"uuid\":\"3b979ad0-f04d-4546-9a99-5921572b1183\"}],\"packageUris\":[\"http://schema.mathworks.com/mf0/Connector/R2020b\"],\"version\":\"1.0\"}"
  Pulmonary Small Veins : Subsystem  Description=asrwer
      settings: PortSchema="{\"entries\":[{\"content\":{\"sides\":[{\"content\":{\"connectorIds\":[\"In1\",\"Out2\"]},\"type\":\"ConnectorPlacement.EquallySpacedRectSide\",\"uuid\":\"4620f5c1-12c0-4f29-952b-739216107ff5\"},{\"content\":{\"connectorIds\":[\"Out1\",\"In2\"],\"side\":\"RIGHT\"},\"type\":\"ConnectorPlacement.EquallySpacedRectSide\",\"uuid\":\"dda98628-74f0-4e08-ba9e-db399286a987\"},{\"content\":{\"connectorIds\":[],\"side\":\"TOP\"},\"type\":\"ConnectorPlacement.EquallySpacedRectSide\",\"uuid\":\"6ce998cb-1877-491b-b2c2-215d41cdcb23\"},{\"content\":{\"connectorIds\":[],\"side\":\"BOTTOM\"},\"type\":\"ConnectorPlacement.EquallySpacedRectSide\",\"uuid\":\"137012d7-11b1-4b2c-ba99-c13cd95b2b50\"}]},\"type\":\"ConnectorPlacement.EquallySpacedConnector\",\"uuid\":\"3b979ad0-f04d-4546-9a99-5921572b1183\"}],\"packageUris\":[\"http://schema.mathworks.com/mf0/Connector/R2020b\"],\"version\":\"1.0\"}"
  Pulmonary Trunk : Subsystem  Description=asrwer
      settings: PortSchema="{\"entries\":[{\"content\":{\"sides\":[{\"content\":{\"connectorIds\":[\"In1\",\"Out2\"]},\"type\":\"ConnectorPlacement.EquallySpacedRectSide\",\"uuid\":\"4620f5c1-12c0-4f29-952b-739216107ff5\"},{\"content\":{\"connectorIds\":[\"Out1\",\"In2\"],\"side\":\"RIGHT\"},\"type\":\"ConnectorPlacement.EquallySpacedRectSide\",\"uuid\":\"dda98628-74f0-4e08-ba9e-db399286a987\"},{\"content\":{\"connectorIds\":[],\"side\":\"TOP\"},\"type\":\"ConnectorPlacement.EquallySpacedRectSide\",\"uuid\":\"6ce998cb-1877-491b-b2c2-215d41cdcb23\"},{\"content\":{\"connectorIds\":[],\"side\":\"BOTTOM\"},\"type\":\"ConnectorPlacement.EquallySpacedRectSide\",\"uuid\":\"04da4d59-f989-4121-a1c1-6ca6c24a4d8d\"}]},\"type\":\"ConnectorPlacement.EquallySpacedConnector\",\"uuid\":\"3b979ad0-f04d-4546-9a99-5921572b1183\"}],\"packageUris\":[\"http://schema.mathworks.com/mf0/Connector/R2020b\"],\"version\":\"1.0\"}"
  Pulmonary Veins : Subsystem  Description=asrwer
      settings: PortSchema="{\"entries\":[{\"content\":{\"sides\":[{\"content\":{\"connectorIds\":[\"In1\",\"Out2\"]},\"type\":\"ConnectorPlacement.EquallySpacedRectSide\",\"uuid\":\"4620f5c1-12c0-4f29-952b-739216107ff5\"},{\"content\":{\"connectorIds\":[\"Out1\",\"In2\"],\"side\":\"RIGHT\"},\"type\":\"ConnectorPlacement.EquallySpacedRectSide\",\"uuid\":\"dda98628-74f0-4e08-ba9e-db399286a987\"},{\"content\":{\"connectorIds\":[],\"side\":\"TOP\"},\"type\":\"ConnectorPlacement.EquallySpacedRectSide\",\"uuid\":\"6ce998cb-1877-491b-b2c2-215d41cdcb23\"},{\"content\":{\"connectorIds\":[],\"side\":\"BOTTOM\"},\"type\":\"ConnectorPlacement.EquallySpacedRectSide\",\"uuid\":\"3a23e96a-9068-4331-9d6b-a32064471a48\"}]},\"type\":\"ConnectorPlacement.EquallySpacedConnector\",\"uuid\":\"3b979ad0-f04d-4546-9a99-5921572b1183\"}],\"packageUris\":[\"http://schema.mathworks.com/mf0/Connector/R2020b\"],\"version\":\"1.0\"}"
  Qaoa delay (s) : EditField  LabelPosition=Hide  ShowInitialText=on  Alignment=Left
  Qpua delay (s) : EditField  LabelPosition=Hide  ShowInitialText=on  Alignment=Left
  RA Emax Gain : EditField  LabelPosition=Hide  ShowInitialText=on  Alignment=Left
  RA Emin Gain : EditField  LabelPosition=Hide  ShowInitialText=on  Alignment=Left
  RV Emax Gain : EditField  LabelPosition=Hide  ShowInitialText=on  Alignment=Left
  RV Emin Gain : EditField  LabelPosition=Hide  ShowInitialText=on  Alignment=Left
  Resistance Arteries : Subsystem  Description=asrwer
      settings: PortSchema="{\"entries\":[{\"content\":{\"sides\":[{\"content\":{\"connectorIds\":[\"In1\",\"Out2\"]},\"type\":\"ConnectorPlacement.EquallySpacedRectSide\",\"uuid\":\"4620f5c1-12c0-4f29-952b-739216107ff5\"},{\"content\":{\"connectorIds\":[\"Out1\",\"In2\"],\"side\":\"RIGHT\"},\"type\":\"ConnectorPlacement.EquallySpacedRectSide\",\"uuid\":\"dda98628-74f0-4e08-ba9e-db399286a987\"},{\"content\":{\"connectorIds\":[],\"side\":\"TOP\"},\"type\":\"ConnectorPlacement.EquallySpacedRectSide\",\"uuid\":\"6ce998cb-1877-491b-b2c2-215d41cdcb23\"},{\"content\":{\"connectorIds\":[],\"side\":\"BOTTOM\"},\"type\":\"ConnectorPlacement.EquallySpacedRectSide\",\"uuid\":\"1ab5c822-e7a5-49ea-823d-95e461b1ff07\"}]},\"type\":\"ConnectorPlacement.EquallySpacedConnector\",\"uuid\":\"3b979ad0-f04d-4546-9a99-5921572b1183\"}],\"packageUris\":[\"http://schema.mathworks.com/mf0/Connector/R2020b\"],\"version\":\"1.0\"}"
  Right Carotid Artery : Subsystem  Description=asrwer
      settings: PortSchema="{\"entries\":[{\"content\":{\"sides\":[{\"content\":{\"connectorIds\":[\"Out2\",\"In1\"]},\"type\":\"ConnectorPlacement.EquallySpacedRectSide\",\"uuid\":\"4620f5c1-12c0-4f29-952b-739216107ff5\"},{\"content\":{\"connectorIds\":[\"Out1\",\"In2\"],\"side\":\"RIGHT\"},\"type\":\"ConnectorPlacement.EquallySpacedRectSide\",\"uuid\":\"dda98628-74f0-4e08-ba9e-db399286a987\"},{\"content\":{\"connectorIds\":[],\"side\":\"TOP\"},\"type\":\"ConnectorPlacement.EquallySpacedRectSide\",\"uuid\":\"6ce998cb-1877-491b-b2c2-215d41cdcb23\"},{\"content\":{\"connectorIds\":[],\"side\":\"BOTTOM\"},\"type\":\"ConnectorPlacement.EquallySpacedRectSide\",\"uuid\":\"5d964695-aedc-48ec-816e-6d149f9baa1a\"}]},\"type\":\"ConnectorPlacement.EquallySpacedConnector\",\"uuid\":\"3b979ad0-f04d-4546-9a99-5921572b1183\"}],\"packageUris\":[\"http://schema.mathworks.com/mf0/Connector/R2020b\"],\"version\":\"1.0\"}"
  Right Carotid Capillaries : Subsystem  Description=asrwer
      settings: PortSchema="{\"entries\":[{\"content\":{\"sides\":[{\"content\":{\"connectorIds\":[\"Out2\",\"In1\"]},\"type\":\"ConnectorPlacement.EquallySpacedRectSide\",\"uuid\":\"4620f5c1-12c0-4f29-952b-739216107ff5\"},{\"content\":{\"connectorIds\":[\"In2\",\"Out1\"],\"side\":\"RIGHT\"},\"type\":\"ConnectorPlacement.EquallySpacedRectSide\",\"uuid\":\"dda98628-74f0-4e08-ba9e-db399286a987\"},{\"content\":{\"connectorIds\":[],\"side\":\"TOP\"},\"type\":\"ConnectorPlacement.EquallySpacedRectSide\",\"uuid\":\"6ce998cb-1877-491b-b2c2-215d41cdcb23\"},{\"content\":{\"connectorIds\":[],\"side\":\"BOTTOM\"},\"type\":\"ConnectorPlacement.EquallySpacedRectSide\",\"uuid\":\"cace3d24-f2c5-4b3d-b351-04ba56070658\"}]},\"type\":\"ConnectorPlacement.EquallySpacedConnector\",\"uuid\":\"3b979ad0-f04d-4546-9a99-5921572b1183\"}],\"packageUris\":[\"http://schema.mathworks.com/mf0/Connector/R2020b\"],\"version\":\"1.0\"}"
  Right Carotid Resistance Artery : Subsystem  Description=asrwer
      settings: PortSchema="{\"entries\":[{\"content\":{\"sides\":[{\"content\":{\"connectorIds\":[\"Out2\",\"In1\"]},\"type\":\"ConnectorPlacement.EquallySpacedRectSide\",\"uuid\":\"4620f5c1-12c0-4f29-952b-739216107ff5\"},{\"content\":{\"connectorIds\":[\"In2\",\"Out1\"],\"side\":\"RIGHT\"},\"type\":\"ConnectorPlacement.EquallySpacedRectSide\",\"uuid\":\"dda98628-74f0-4e08-ba9e-db399286a987\"},{\"content\":{\"connectorIds\":[],\"side\":\"TOP\"},\"type\":\"ConnectorPlacement.EquallySpacedRectSide\",\"uuid\":\"6ce998cb-1877-491b-b2c2-215d41cdcb23\"},{\"content\":{\"connectorIds\":[],\"side\":\"BOTTOM\"},\"type\":\"ConnectorPlacement.EquallySpacedRectSide\",\"uuid\":\"f6d8c471-30f5-492c-bb7b-f051effd3cec\"}]},\"type\":\"ConnectorPlacement.EquallySpacedConnector\",\"uuid\":\"3b979ad0-f04d-4546-9a99-5921572b1183\"}],\"packageUris\":[\"http://schema.mathworks.com/mf0/Connector/R2020b\"],\"version\":\"1.0\"}"
  Right Carotid Vein : Subsystem  Description=asrwer
      settings: PortSchema="{\"entries\":[{\"content\":{\"sides\":[{\"content\":{\"connectorIds\":[\"Out2\",\"In1\"]},\"type\":\"ConnectorPlacement.EquallySpacedRectSide\",\"uuid\":\"4620f5c1-12c0-4f29-952b-739216107ff5\"},{\"content\":{\"connectorIds\":[\"In2\",\"Out1\"],\"side\":\"RIGHT\"},\"type\":\"ConnectorPlacement.EquallySpacedRectSide\",\"uuid\":\"dda98628-74f0-4e08-ba9e-db399286a987\"},{\"content\":{\"connectorIds\":[],\"side\":\"TOP\"},\"type\":\"ConnectorPlacement.EquallySpacedRectSide\",\"uuid\":\"6ce998cb-1877-491b-b2c2-215d41cdcb23\"}]},\"type\":\"ConnectorPlacement.EquallySpacedConnector\",\"uuid\":\"3b979ad0-f04d-4546-9a99-5921572b1183\"}],\"packageUris\":[\"http://schema.mathworks.com/mf0/Connector/R2020b\"],\"version\":\"1.0\"}"
  SAP measured : DisplayBlock  LabelPosition=Hide  Format=Custom  Alignment=Left  Transparency=1  Layout=Fill available space  FormatString=%.2f
  SAP target : EditField  LabelPosition=Hide  ShowInitialText=on  Alignment=Left
  SAP/DAP control : Vessel/SAP//DAP control  SAP_0=SAP  DAP_0=DAP  dt=0.1  onoff=off
      link override Constant1: Value=0
      link override K_Y_aorta: Value=0
      link override K_Y_systemic_veins: Value=0
      link override PID Controller: UpperSaturationLimit=5
      settings: SourceProductName=CVM
  "SAP/DAP control " : SliderSwitchBlock  LabelPosition=Hide
      settings: Values={{'Off', 'On'}, [0 1]}
  SLVP control : Vessel/SLVP control  SLVP_0=MAP  dt=1  onoff=off
      link override Constant1: Value=0
      link override K_LA_Emax: Value=0
      link override K_LA_Emin: Value=0
      link override K_LV_Emax: Value=0
      link override K_LV_Emin: Value=0
      link override PID Controller: P=0.01  I=0.01  UpperSaturationLimit=5
      settings: LibrarySourceBlock=Vessel/SAP control  SourceProductName=CVM
  "SLVP control  " : SliderSwitchBlock  LabelPosition=Hide
      settings: Values={{'Off', 'On'}, [0 1]}
  SLVP measured : DisplayBlock  LabelPosition=Hide  Format=Custom  Alignment=Left  Transparency=1  Layout=Fill available space  FormatString=%.2f
  SLVP target : EditField  LabelPosition=Hide  ShowInitialText=on  Alignment=Left
  SPP measured : DisplayBlock  LabelPosition=Hide  Format=Custom  Alignment=Left  Transparency=1  Layout=Fill available space  FormatString=%.2f
  SPP target : EditField  LabelPosition=Hide  ShowInitialText=on  Alignment=Left
  SPP/DPP control : Vessel/SPP//DPP control  SPP_0=SPP  DPP_0=DPP  dt=0.1  onoff=off
      link override Constant1: Value=0
      link override K_Y_pulmonary_arteries: Value=0
      link override K_Y_pulmonary_veins: Value=0
      link override PID Controller: P=0.01  I=0.01  UpperSaturationLimit=5
      settings: SourceProductName=CVM
  "SPP/DPP control " : SliderSwitchBlock  LabelPosition=Hide
      settings: Values={{'Off', 'On'}, [0 1]}
  SRVP control : Vessel/SRVP control  SRVP_0=MPP  dt=1  onoff=off
      link override Constant1: Value=0
      link override K_RA_Emax: Value=0
      link override K_RA_Emin: Value=0
      link override K_RV_Emax: Value=0
      link override K_RV_Emin: Value=0
      link override PID Controller: P=0.01  I=0.01  UpperSaturationLimit=6
      settings: LibrarySourceBlock=Vessel/SPP control1  SourceProductName=CVM
  "SRVP control " : SliderSwitchBlock  LabelPosition=Hide
      settings: Values={{'Off', 'On'}, [0 1]}
  SRVP measured : DisplayBlock  LabelPosition=Hide  Format=Custom  Alignment=Left  Transparency=1  Layout=Fill available space  FormatString=%.2f
  SRVP target : EditField  LabelPosition=Hide  ShowInitialText=on  Alignment=Left
  SVR (mmHg s / ml) : DisplayBlock  LabelPosition=Hide  Format=Custom  Alignment=Left  Transparency=1  Layout=Fill available space  FormatString=%.2f
  SVR Control : Vessel/SVR Control  SVR_0=SVR  onoff=off
      link override Constant1: Value=0
      link override K_svr: Value=0
      settings: SourceProductName=CVM
  SVR Gain : EditField  LabelPosition=Hide  ShowInitialText=on  Alignment=Left
  SVR control : SliderSwitchBlock  LabelPosition=Hide
      settings: Values={{'Off', 'On'}, [0 1]}
  SVR measured : DisplayBlock  LabelPosition=Hide  Format=Custom  Alignment=Left  Transparency=1  Layout=Fill available space  FormatString=%.2f
  SVR target : EditField  LabelPosition=Hide  ShowInitialText=on  Alignment=Left
  Stroke Volume (ml) : DisplayBlock  LabelPosition=Hide  Format=Custom  Alignment=Left  Transparency=1  Layout=Fill available space  FormatString=%.2f
  Subtract2 : Sum  Inputs=-+
  Subtract3 : Sum  Inputs=+-
  Subtract4 : Sum
  Subtract5 : Sum
  Superior Caval Vein : Subsystem  Description=asrwer
      settings: PortSchema="{\"entries\":[{\"content\":{\"sides\":[{\"content\":{\"connectorIds\":[\"In1\",\"Out2\"]},\"type\":\"ConnectorPlacement.EquallySpacedRectSide\",\"uuid\":\"4620f5c1-12c0-4f29-952b-739216107ff5\"},{\"content\":{\"connectorIds\":[\"In2\",\"Out1\"],\"side\":\"RIGHT\"},\"type\":\"ConnectorPlacement.EquallySpacedRectSide\",\"uuid\":\"dda98628-74f0-4e08-ba9e-db399286a987\"},{\"content\":{\"connectorIds\":[],\"side\":\"TOP\"},\"type\":\"ConnectorPlacement.EquallySpacedRectSide\",\"uuid\":\"6ce998cb-1877-491b-b2c2-215d41cdcb23\"},{\"content\":{\"connectorIds\":[],\"side\":\"BOTTOM\"},\"type\":\"ConnectorPlacement.EquallySpacedRectSide\",\"uuid\":\"5f47a899-ed05-43b2-ba58-6d035433b88e\"}]},\"type\":\"ConnectorPlacement.EquallySpacedConnector\",\"uuid\":\"3b979ad0-f04d-4546-9a99-5921572b1183\"}],\"packageUris\":[\"http://schema.mathworks.com/mf0/Connector/R2020b\"],\"version\":\"1.0\"}"
  "Systemic Capillaries " : Subsystem  Description=asrwer
      settings: PortSchema="{\"entries\":[{\"content\":{\"sides\":[{\"content\":{\"connectorIds\":[\"In1\",\"Out2\"]},\"type\":\"ConnectorPlacement.EquallySpacedRectSide\",\"uuid\":\"4620f5c1-12c0-4f29-952b-739216107ff5\"},{\"content\":{\"connectorIds\":[\"In2\",\"Out1\"],\"side\":\"RIGHT\"},\"type\":\"ConnectorPlacement.EquallySpacedRectSide\",\"uuid\":\"dda98628-74f0-4e08-ba9e-db399286a987\"},{\"content\":{\"connectorIds\":[],\"side\":\"TOP\"},\"type\":\"ConnectorPlacement.EquallySpacedRectSide\",\"uuid\":\"6ce998cb-1877-491b-b2c2-215d41cdcb23\"},{\"content\":{\"connectorIds\":[],\"side\":\"BOTTOM\"},\"type\":\"ConnectorPlacement.EquallySpacedRectSide\",\"uuid\":\"621182d5-32aa-4c84-a747-47e09e96be96\"}]},\"type\":\"ConnectorPlacement.EquallySpacedConnector\",\"uuid\":\"3b979ad0-f04d-4546-9a99-5921572b1183\"}],\"packageUris\":[\"http://schema.mathworks.com/mf0/Connector/R2020b\"],\"version\":\"1.0\"}"
  Systolic : DisplayBlock  LabelPosition=Hide  Format=Custom  Alignment=Left  Transparency=1  Layout=Fill available space  FormatString=%.2f
  Total Blood Volume : Subsystem
  UVV (ml) : DisplayBlock  LabelPosition=Hide  Format=Custom  Alignment=Left  Transparency=1  Layout=Fill available space  FormatString=%.2f
  UVV Control : Vessel/UVV Control  UVV_0=UVV  onoff=off
      link override Constant1: Value=0
      link override K_uvv: Value=0
      link override PID Controller: I=0.001
      link override PID Controller1: LowerSaturationLimit=-0.95  P=0.001  I=0.001
      settings: SourceProductName=CVM
  UVV Gain : EditField  LabelPosition=Hide  ShowInitialText=on  Alignment=Left
  UVV control : SliderSwitchBlock  LabelPosition=Hide
      settings: Values={{'Off', 'On'}, [0 1]}
  UVV measured : DisplayBlock  LabelPosition=Hide  Format=Custom  Alignment=Left  Transparency=1  Layout=Fill available space  FormatString=%.2f
  UVV target : EditField  LabelPosition=Hide  ShowInitialText=on  Alignment=Left
  Ventricle (Peak) : DisplayBlock  LabelPosition=Hide  Format=Custom  Alignment=Left  Transparency=1  Layout=Fill available space  FormatString=%.2f
  Y pul art Gain : EditField  LabelPosition=Hide  ShowInitialText=on  Alignment=Left
  Y pul veins Gain : EditField  LabelPosition=Hide  ShowInitialText=on  Alignment=Left
  Y sys art Gain : EditField  LabelPosition=Hide  ShowInitialText=on  Alignment=Left
  Y sys veins Gain : EditField  LabelPosition=Hide  ShowInitialText=on  Alignment=Left
  Aorta (ascending) : Scope
  Aorta (descending) : Scope
  Aorta (distal) : Scope
  Aorta (proxima) : Scope
  Aorta (root) : Scope
  Aortic Valve : Scope
  Aplysia graphs : Scope
  Baroflex control : Scope
  Cardiac Output control : Scope
  Carotid Artery (left) : Scope
  Carotid Artery (right) : Scope
  Carotid Capillaries (left) : Scope
  Carotid Capillaries (right) : Scope
  Carotid resistance Artery (right) : Scope
  Carotid veins (right) : Scope
  Coronary Resistance Artery (right) : Scope
  Coronary arteries flow : Scope
  Elastances : Scope
  Heart Pressures : Scope
  Heart Volume : Scope
  Impedance convergence : Scope
  Inferior Vena cava : Scope
  Intrathoracic pressure : Scope
  Left ventricle/Aortic Pressure : Scope
  Mitral Valve : Scope
  Pressure Wave Propagation : Scope
  Pulmonary Valve : Scope
  Pulmonary capillaries : Scope
  R/ Atrium : Scope
  Scope{,1..6} (7 alike) : Scope
  Superior Vena cava : Scope
  Sys perifereal arteries : Scope
  Sys resistance arteries : Scope
  Systemic Capillaries : Scope
  Systemic Veins : Scope
  Total Bloob Volume : Scope
  Tricuspid Valve : Scope
  Ved : Scope
  Venous return : Scope
  wires:
  Pulmonary Trunk/2("Q_Output ") -> Pulmonary Arteries/1(Q_Input)
  Pulmonary Arteries/2("P_Input ") -> Pulmonary Trunk/1(P_Output)
  Pulmonary Arteries/1("Q_Output ") -> Pulmonary Resistance Arteries/1(Q_Input)
  Pulmonary Resistance Arteries/2("P_Input ") -> Pulmonary Arteries/2(P_Output)
  Pulmonary Resistance Arteries/1("Q_Output ") -> Pulmonary Capillaries/1(Q_Input)
  Pulmonary Capillaries/2("P_Input ") -> Pulmonary Resistance Arteries/2(P_Output)
  Pulmonary Capillaries/1("Q_Output ") -> Pulmonary Small Veins/1(Q_Input)
  Pulmonary Small Veins/2("P_Input ") -> Pulmonary Capillaries/2(P_Output)
  Pulmonary Small Veins/1("Q_Output ") -> Pulmonary Veins/1(Q_Input)
  Pulmonary Veins/2("P_Input ") -> Pulmonary Small Veins/2(P_Output)
  Aortic root/1("Q_Output ") -> Ascending aorta/2(Q_Input)
  Ascending aorta/1("P_Input ") -> Aortic root/2(P_Output)
  Ascending aorta/2("Q_Output ") -> Subtract2/2
  Proximal aortic arch/2("P_Input ") -> Ascending aorta/1(P_Output), Right Carotid Artery/2(P_Input)
  Proximal aortic arch/1("Q_Output ") -> Subtract3/1
  Distal aortic arch/2("Q_Output ") -> Descending aorta/2(Q_Input)
  Descending aorta/1("P_Input ") -> Distal aortic arch/1(P_Output)
  Peripheral Arteries/1("P_Input ") -> Descending aorta/1(P_Output)
  Descending aorta/2("Q_Output ") -> Peripheral Arteries/2(Q_Input)
  Peripheral Arteries/2("Q_Output ") -> Resistance Arteries/1(Q_Input)
  Resistance Arteries/2("P_Input ") -> Peripheral Arteries/1(P_Output)
  Resistance Arteries/1("Q_Output ") -> "Systemic Capillaries "/2(Q_Input)
  "Systemic Capillaries "/1("P_Input ") -> Resistance Arteries/2(P_Output)
  "Systemic Capillaries "/2("Q_Output ") -> Capacitance Vessels/1(Q_Input)
  Capacitance Vessels/2("P_Input ") -> "Systemic Capillaries "/1(P_Output)
  Inferior Caval Vein/1("P_Input ") -> Capacitance Vessels/2(P_Output)
  Capacitance Vessels/1("Q_Output ") -> Inferior Caval Vein/1(Q_Input)
  Right Carotid Artery/1(Q_Input) -> Subtract2/1
  Subtract2/1 -> Proximal aortic arch/1(Q_Input)
  Subtract3/1 -> Distal aortic arch/2(Q_Input)
  Left Carotid Artery/1(Q_Input) -> Subtract3/2
  Distal aortic arch/1("P_Input ") -> Proximal aortic arch/2(P_Output), Left Carotid Artery/2(P_Input)
  Left Carotid Capillaries/2(Q_Out) -> Left Carotid Vein/2(Q_Input)
  Left Carotid Vein/1("P_Input ") -> Left Carotid Capillaries/1(P_Output)
  Right Carotid Capillaries/2(Q_Out) -> Right Carotid Vein/2(Q_Input)
  Right Carotid Vein/1("P_Input ") -> Right Carotid Capillaries/1(P_Output)
  Superior Caval Vein/2("P_Input ") -> Left Carotid Vein/1(P_Output), Right Carotid Vein/1(P_Output)
  Subtract4/1 -> Superior Caval Vein/1(Q_Input)
  Right Carotid Vein/2("Q_Output ") -> Subtract4/2
  Left Carotid Vein/2("Q_Output ") -> Subtract4/1
  Inferior Caval Vein/2("Q_Output ") -> Subtract5/2
  Superior Caval Vein/1("Q_Output ") -> Subtract5/1
  Subtract5/1 -> Heart/2(Q_Ra)
  Heart/3(Q_pul) -> Pulmonary Trunk/2(Q_Input)
  Heart/2(Q_aor) -> Aortic root/1(Q_Input)
  Aortic root/2("P_Input ") -> Heart/4(P_aor)
  Pulmonary Trunk/1("P_Input ") -> Heart/1(P_pul)
  Pulmonary Veins/1("Q_Output ") -> Heart/3(Q_La)
  Heart/1(P_La) -> Pulmonary Veins/2(P_Output)
  Heart/4(P_Ra) -> Superior Caval Vein/2(P_Output), Inferior Caval Vein/2(P_Output)
  Left Carotid Capillaries/1(P_input) -> Left Carotid Resistance Artery/1(P_Output)
  Left Carotid Resistance Artery/2(Q_Output) -> Left Carotid Capillaries/2(Q_Input)
  Right Carotid Resistance Artery/2(Q_Output) -> Right Carotid Capillaries/2(Q_Input1)
  Right Carotid Capillaries/1(P_input) -> Right Carotid Resistance Artery/1(P_Output)
  Right Carotid Artery/2(Q_Output) -> Right Carotid Resistance Artery/2(Q_Input1)
  Right Carotid Resistance Artery/1(P_input) -> Right Carotid Artery/1(P_Output)
  Left Carotid Artery/2(Q_Output) -> Left Carotid Resistance Artery/2(Q_Input1)
  Left Carotid Resistance Artery/1(P_input) -> Left Carotid Artery/1(P_Output)
  Constant/1 -> Data Store Write/1
  [P_sys] -> Display/1
